simulink model "DC_Supply_Arch"  (R2022b)
settings: Solver=FixedStepDiscrete  StartTime=0.0  StopTime=10.0  RelTol=1e-3
settings Model: Creator=MAAM  LastModifiedBy=MAAM

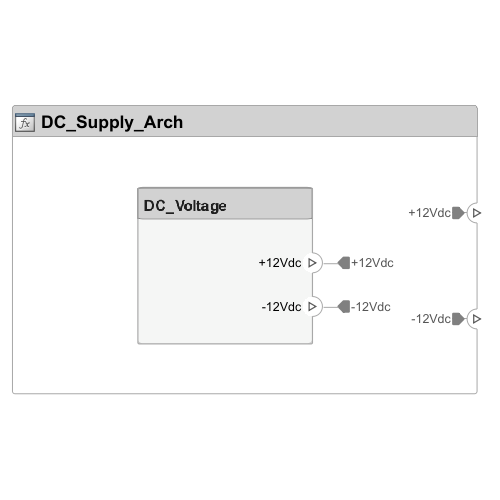
[thumbnail: Simulink's stored preview of the top-level diagram]
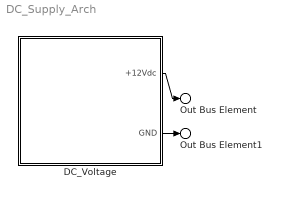
== system DC_Supply_Arch ==
  DC_Voltage : Subsystem
      settings: PortSchema="{\"entries\":[{\"content\":{\"headerSize\":26,\"margin\":15,\"minimumSpacing\":25,\"sides\":[{\"content\":{\"connectorIds\":[]},\"type\":\"ConnectorPlacement.EquallySpacedRectSide\",\"uuid\":\"ecb73a61-b18a-4e6f-9a16-a7412467d3dc\"},{\"content\":{\"connectorIds\":[\"Out1\",\"Out2\"],\"side\":\"RIGHT\"},\"type\":\"ConnectorPlacement.EquallySpacedRectSide\",\"uuid\":\"05d75da6-23d5-4864-9569-f2b0c11a82bb\"},{\"content\":{\"connectorIds\":[],\"side\":\"TOP\"},\"type\":\"ConnectorPlacement.EquallySpacedRectSide\",\"uuid\":\"f7c561b3-9491-4c59-9ccb-7eaec9c6a3d8\"}]},\"type\":\"ConnectorPlacement.EquallySpacedConnector\",\"uuid\":\"7fcac072-6609-4f2b-820d-d62cc0efbf31\"}],\"packageUris\":[\"http://schema.mathworks.com/mf0/Connector/R2020b\"],\"version\":\"1.0\"}"
  Out Bus Element : Outport  PortName=+12Vdc
  Out Bus Element1 : Outport  Port=2  PortName=GND
  wires:
  DC_Voltage/1(+12Vdc) -> Out Bus Element/1
  DC_Voltage/2(GND) -> Out Bus Element1/1

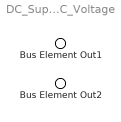
== system DC_Supply_Arch/DC_Voltage ==
  Bus Element Out1 : Outport  PortName=+12Vdc
  Bus Element Out2 : Outport  Port=2  PortName=GND
